simulink model "Elevator"  (R2022a)
settings: Solver=VariableStepAuto  StartTime=0.0  StopTime=inf  RelTol=1e-3
settings Model: Creator=Amogh  LastModifiedBy=Amogh

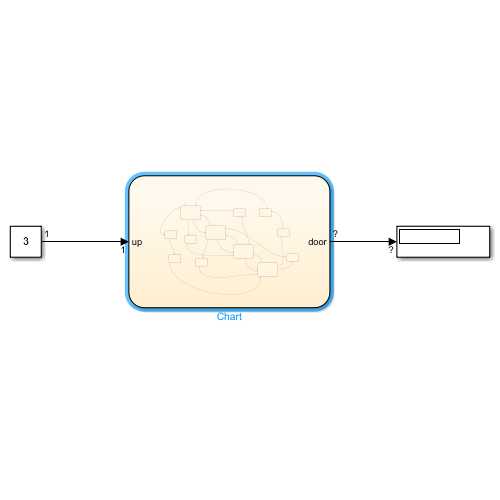
[thumbnail: Simulink's stored preview of the top-level diagram]
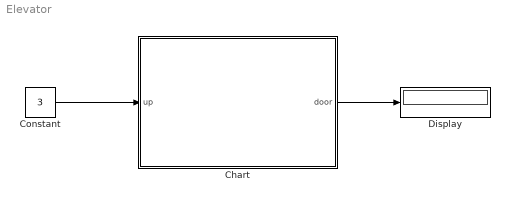
== system Elevator ==
  Chart : Stateflow chart  TreatAsAtomicUnit=on
  Constant : Constant  Value=3
  Display : Display
  wires:
  Constant/1 -> Chart/1(up)
  Chart/1(door) -> Display/1

== stateflow chart Elevator/Chart ==
  state Ground_F
    entry:
    door=1;
    exit:
    door=0;
  state skipfirst3
    entry:
    door=0;
  state skipfirst5
    entry:
    door=0;
  state First_F
    entry:
    door=1;
    exit:
    door=0;
  state skipsecond4
    entry:
    door=0;
  state skipfirst2
    entry:
    door=0;
  state skipfirst1
    entry:
    door=0;
  state Second_F
    entry:
    door=1;
    exit:
    door=0;
  state skipsecond3
    entry:
    door=0;
  state skipsecond2
    entry:
    door=0;
  state skipsecond1
    entry:
    door=0;
  state Third_F
    entry:
    door=1;
    exit:
    door=0;
  skipfirst5 -> Ground_F
  (default) -> Ground_F
  Ground_F -> skipfirst2 [order 3] : [up==3]
  skipfirst3 -> Ground_F
  skipsecond4 -> skipfirst5
  First_F -> Ground_F [order 1] : [up==0]
  Second_F -> skipfirst3 [order 3] : [up==0]
  Ground_F -> skipfirst1 [order 2] : [up==2]
  Ground_F -> First_F [order 1] : [up==1]
  skipsecond3 -> First_F
  Second_F -> First_F [order 1] : [up==1]
  Third_F -> skipsecond4 [order 3] : [up==0]
  skipfirst2 -> skipsecond2
  First_F -> skipsecond1 [order 3] : [up==3]
  First_F -> Second_F [order 2] : [up==2]
  skipfirst1 -> Second_F
  Third_F -> Second_F [order 1] : [up==2]
  Second_F -> Third_F [order 2] : [up==3]
  Third_F -> skipsecond3 [order 2] : [up==1]
  skipsecond2 -> Third_F
  skipsecond1 -> Third_F
  data: door output; up input
